simulink model "ampc_cstr_lpv"  (R2021a)
settings: Solver=ode45  StartTime=0.0  StopTime=400
undefined symbols (not defined in the file or in its folder): sigbuilder_block
libraries: mpclib x1, cstblocks x1, simulink x1
settings Model: Creator=Oluwatofunmi  LastModifiedBy=USER
settings SolverCC: AlgebraicLoopSolver=TrustRegion
settings DebuggingCC: PregeneratedLibrarySubsystemCodeDiagnostic=none  SFMachineParentedDataDiag=warning  ArithmeticOperatorsInVariantConditions=warning
settings SFSimCC: CustomCodeUndefinedFunction=UseInterfaceOnly

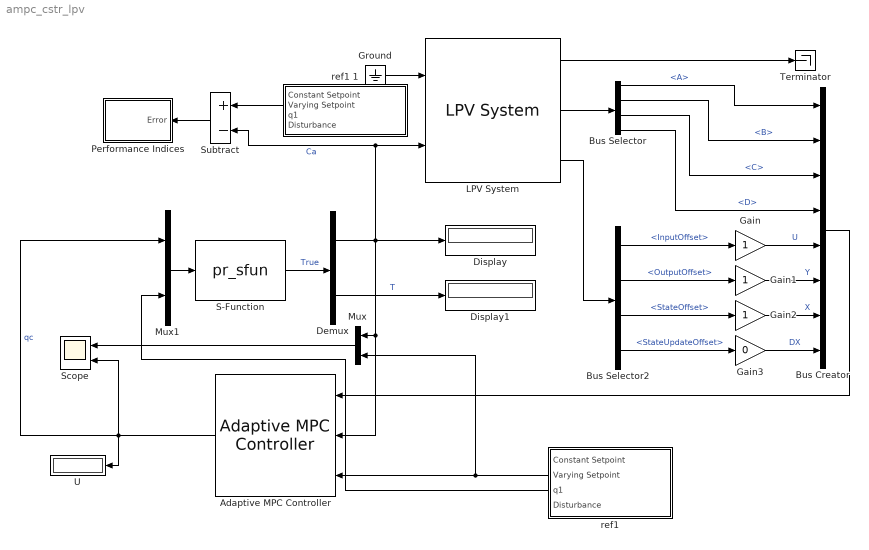
== system ampc_cstr_lpv ==
  Adaptive MPC Controller : mpclib/Adaptive MPC Controller  SCDEnableBlockLinearizationSpecification=on  mpcobj=mpcobj_lpv  enable_value=0  updateMPCinCallerWorkspace=on  md_inport=off  mv_inport=off  uref_inport=off  return_cost=off  return_mvseq=off  return_qpstatus=off  return_xseq=off  return_state=off  return_ovseq=off  state_inport=off  isltv_plant=off  umin_inport=off  umax_inport=off  ymin_inport=off  ymax_inport=off  cc_inport=off  ywt_inport=off  uwt_inport=off  duwt_inport=off  rhoeps_inport=off  pm_inport=off  MaximumP=10  HorizonChoice=FixedHorizon  BlockDataType=double  SampleTimeInherited=off  switch_inport=off
  Bus Creator : BusCreator  Inputs=8
  Bus Selector : BusSelector  OutputSignals=A,B,C,D
  Bus Selector2 : BusSelector  OutputSignals=InputOffset,OutputOffset,StateOffset,StateUpdateOffset
  Demux : Demux  Outputs=2
  Display : Display
  Display1 : Display
  Gain : Gain
  Gain1 : Gain
  Gain2 : Gain
  Gain3 : Gain  Gain=0
  Ground : Ground
  LPV System : cstblocks/Linear Parameter Varying/LPV System  sys=lpv  x0=0  uOffset=lpv_u0  yOffset=lpv_y0  xOffset=lpv_x0  opEquilOption=on  dxOffset=0  sysFixedOption=Use the first model in state-space array  sysFixed=[]  AFixed=false  BFixed=false  CFixed=false  DFixed=false  uDelayFixed=true  yDelayFixed=true  iDelayFixed=true  IMethod=Linear  EMethod=Clip  IndexSearch=Binary search  IndexBegin=on  OutputX=off  OutputXdot=off  OutputLTI=on  OutputOP=on  DataType=double  SimMode=Interpreted execution  InitBufferSize=1024  FixedBuffer=off
      settings: SourceProductBaseCode=CT
  Mux : Mux  Inputs=2
  Mux1 : Mux  Inputs=2
  Performance Indices : Subsystem
  S-Function : S-Function  FunctionName=pr_sfun  SFunctionDeploymentMode=off  EnableBusSupport=off
  Scope : Scope  NumInputPorts=2
  Subtract : Sum  Inputs=+-
  Terminator : Terminator
  U : Display
  "ref1 " : Subsystem  Tag=STV Subsys  LoadFcn=sigbuilder_block('load');  StartFcn=sigbuilder_block('start');  StopFcn=sigbuilder_block('stop');  ClipboardFcn=sigbuilder_block('clipboard');  mask(Sigbuilder block){tuvar=[0:10]}
      mask help: Simulink:masks:SigbuilderBlock_MD
      mask init:
      | if ~strcmp(get_param(bdroot(gcbh),'SimulationStatus'),'stopped') tuvar = sigbuilder_block('maskInit'); end
      settings: CopyFcn=sigbuilder_block('copy');  DeleteFcn=sigbuilder_block('delete');  ModelCloseFcn=sigbuilder_block('modelClose');  PreSaveFcn=sigbuilder_block('preSave');  PauseFcn=sigbuilder_block('pause');  ContinueFcn=sigbuilder_block('continue');  NameChangeFcn=sigbuilder_block('namechange');  OpenFcn=sigbuilder_block('open',[5.5 0 949 448 ]);  CloseFcn=sigbuilder_block('close');
      mask Display: plot(0, 0, 100, 100,[2, 2, 32, 32, 2], [68, 8, 8, 68, 68],[32, 2], [38, 38], [32, 19, 2],[53, 60, 44], [32, 17, 17, 2],[16, 16, 31, 31]);txt = getActiveGroup(gcbh);text(2, 100, txt,'verticalAlignment', 'top');
  ref1 1 : Subsystem  Tag=STV Subsys  LoadFcn=sigbuilder_block('load');  StartFcn=sigbuilder_block('start');  StopFcn=sigbuilder_block('stop');  ClipboardFcn=sigbuilder_block('clipboard');  mask(Sigbuilder block){tuvar=[0:10]}
      mask help: Simulink:masks:SigbuilderBlock_MD
      mask init:
      | if ~strcmp(get_param(bdroot(gcbh),'SimulationStatus'),'stopped') tuvar = sigbuilder_block('maskInit'); end
      settings: CopyFcn=sigbuilder_block('copy');  DeleteFcn=sigbuilder_block('delete');  ModelCloseFcn=sigbuilder_block('modelClose');  PreSaveFcn=sigbuilder_block('preSave');  PauseFcn=sigbuilder_block('pause');  ContinueFcn=sigbuilder_block('continue');  NameChangeFcn=sigbuilder_block('namechange');  OpenFcn=sigbuilder_block('open',[5.5 0 949 448 ]);  CloseFcn=sigbuilder_block('close');
      mask Display: plot(0, 0, 100, 100,[2, 2, 32, 32, 2], [68, 8, 8, 68, 68],[32, 2], [38, 38], [32, 19, 2],[53, 60, 44], [32, 17, 17, 2],[16, 16, 31, 31]);txt = getActiveGroup(gcbh);text(2, 100, txt,'verticalAlignment', 'top');
  wires:
  Mux/1 -> Scope/1
  "ref1 "/2(Varying Setpoint) -> Adaptive MPC Controller/3, Mux/2
  Subtract/1 -> Performance Indices/1(Error)
  ref1 1/2(Varying Setpoint) -> Subtract/1
  Demux/1 -> Subtract/2, LPV System/2, Display/1, Adaptive MPC Controller/2, Mux/1  "Ca"
  Demux/2 -> Display1/1  "T"
  S-Function/1 -> Demux/1  "True"
  "ref1 "/3(q1) -> Mux1/2
  Mux1/1 -> S-Function/1
  Bus Selector2/3 -> Gain2/1  "<StateOffset>"
  Bus Selector2/4 -> Gain3/1  "<StateUpdateOffset>"
  LPV System/1 -> Terminator/1
  Gain1/1 -> Bus Creator/6  "Y"
  Bus Selector2/2 -> Gain1/1  "<OutputOffset>"
  Gain3/1 -> Bus Creator/8  "DX"
  LPV System/3 -> Bus Selector2/1
  Gain/1 -> Bus Creator/5  "U"
  Bus Creator/1 -> Adaptive MPC Controller/1
  Ground/1 -> LPV System/1
  Bus Selector2/1 -> Gain/1  "<InputOffset>"
  LPV System/2 -> Bus Selector/1
  Gain2/1 -> Bus Creator/7  "X"
  Bus Selector/4 -> Bus Creator/4  "<D>"
  Bus Selector/3 -> Bus Creator/3  "<C>"
  Bus Selector/1 -> Bus Creator/1  "<A>"
  Bus Selector/2 -> Bus Creator/2  "<B>"
  Adaptive MPC Controller/1 -> Mux1/1, Scope/2, U/1  "qc"

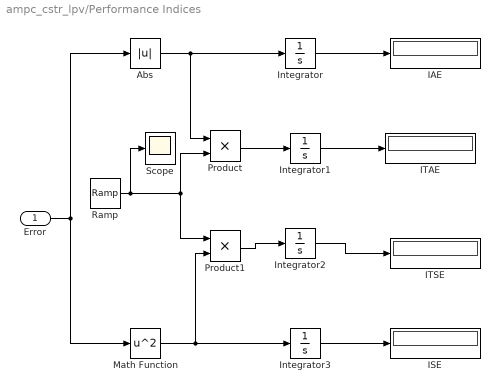
== system ampc_cstr_lpv/Performance Indices ==
  Error : Inport
  Abs : Abs
  IAE : Display
  ISE : Display
  ITAE : Display
  ITSE : Display
  Integrator{,1..3} (4 alike) : Integrator
  Math Function : Math  Operator=square  SignedPower=on  SaturateOnIntegerOverflow=on
  Product : Product  RndMeth=Zero
  Product1 : Product  RndMeth=Zero
  Ramp : simulink/Sources/Ramp  slope=1  start=0  InitialOutput=0
  Scope : Scope
  wires:
  Error/1 -> Math Function/1, Abs/1
  Abs/1 -> Integrator/1, Product/1
  Integrator/1 -> IAE/1
  Ramp/1 -> Product/2, Product1/1, Scope/1
  Math Function/1 -> Integrator3/1, Product1/2
  Product1/1 -> Integrator2/1
  Product/1 -> Integrator1/1
  Integrator3/1 -> ISE/1
  Integrator2/1 -> ITSE/1
  Integrator1/1 -> ITAE/1

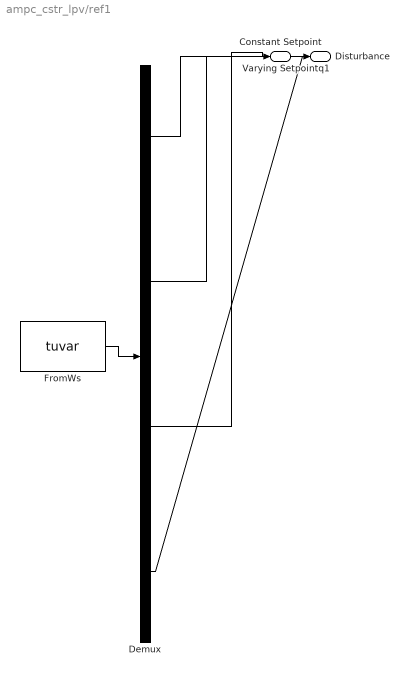
== system ampc_cstr_lpv/ref1  ==
  Demux : Demux  Tag=STV Demux
      settings: DisplayOption=none
  FromWs : FromWorkspace  Tag=STV FromWs  VariableName=tuvar
      SigBuilderData=|
      | common.afterFinalStr = 'Extrapolate'
      | common.sampleTime = 0
      | dataSet.timeRange = [0 400]
      | dataSet.name = 'Group 1'
      | sbobj.Groups.Name = 'Group 1'
      | sbobj.Groups.Signals(1).Name = 'Constant Setpoint'
      | sbobj.Groups.Signals(1).XData = [0 400]
      | sbobj.Groups.Signals(1).YData = [0.1 0.1]
      | sbobj.Groups.Signals(2).Name = 'Varying Setpoint'
      | sbobj.Groups.Signals(2).XData = [0 50 50 150 150 300 300 400]
      | sbobj.Groups.Signals(2).YData = [0.085 0.085 0.1 0.1 0.04 0.04 0.1 0.1]
      | sbobj.Groups.Signals(3).Name = 'q1'
      | sbobj.Groups.Signals(3).XData = [0 400]
      | sbobj.Groups.Signals(3).YData = [100 100]
      | sbobj.Groups.Signals(4).Name = 'Disturbance'
      | sbobj.Groups.Signals(4).XData = [0 50 50 150 150 300 300 400]
      | sbobj.Groups.Signals(4).YData = [100 100 95 95 105 105 100 100]
      | sbobj.Groups.TimeRange = [0 400]
  Constant Setpoint : Outport  Tag=STV Outport
  Varying Setpoint : Outport  Tag=STV Outport  Port=2  VectorParamsAs1DForOutWhenUnconnected=off
  q1 : Outport  Tag=STV Outport  Port=3
  Disturbance : Outport  Tag=STV Outport  Port=4
  wires:
  FromWs/1 -> Demux/1
  Demux/1 -> Constant Setpoint/1
  Demux/2 -> Varying Setpoint/1
  Demux/3 -> q1/1
  Demux/4 -> Disturbance/1

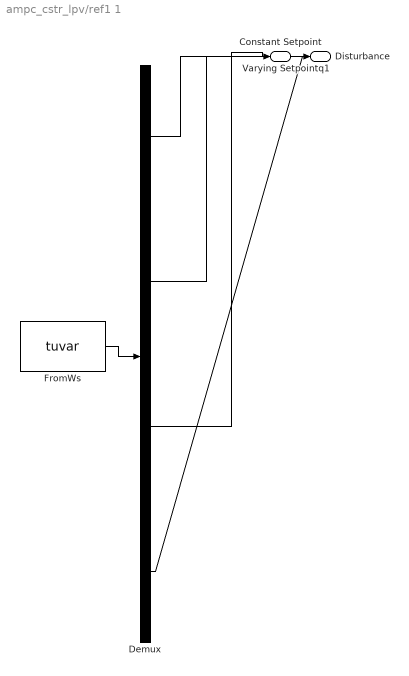
== system ampc_cstr_lpv/ref1 1 ==
  Demux : Demux  Tag=STV Demux
      settings: DisplayOption=none
  FromWs : FromWorkspace  Tag=STV FromWs  VariableName=tuvar
      SigBuilderData=|
      | common.afterFinalStr = 'Extrapolate'
      | common.sampleTime = 0
      | dataSet.timeRange = [0 400]
      | dataSet.name = 'Group 1'
      | sbobj.Groups.Name = 'Group 1'
      | sbobj.Groups.Signals(1).Name = 'Constant Setpoint'
      | sbobj.Groups.Signals(1).XData = [0 400]
      | sbobj.Groups.Signals(1).YData = [0.1 0.1]
      | sbobj.Groups.Signals(2).Name = 'Varying Setpoint'
      | sbobj.Groups.Signals(2).XData = [0 50 50 150 150 300 300 400]
      | sbobj.Groups.Signals(2).YData = [0.085 0.085 0.1 0.1 0.04 0.04 0.1 0.1]
      | sbobj.Groups.Signals(3).Name = 'q1'
      | sbobj.Groups.Signals(3).XData = [0 400]
      | sbobj.Groups.Signals(3).YData = [100 100]
      | sbobj.Groups.Signals(4).Name = 'Disturbance'
      | sbobj.Groups.Signals(4).XData = [0 50 50 150 150 300 300 400]
      | sbobj.Groups.Signals(4).YData = [100 100 95 95 105 105 100 100]
      | sbobj.Groups.TimeRange = [0 400]
  Constant Setpoint : Outport  Tag=STV Outport
  Varying Setpoint : Outport  Tag=STV Outport  Port=2  VectorParamsAs1DForOutWhenUnconnected=off
  q1 : Outport  Tag=STV Outport  Port=3
  Disturbance : Outport  Tag=STV Outport  Port=4
  wires:
  FromWs/1 -> Demux/1
  Demux/1 -> Constant Setpoint/1
  Demux/2 -> Varying Setpoint/1
  Demux/3 -> q1/1
  Demux/4 -> Disturbance/1
